simulink model "glucagon_model_ins"  (R2023b)
settings: Solver=VariableStepAuto  StartTime=0.0  StopTime=300  RelTol=1e-3
values from neighbouring files (symbols this model uses):
  GLUCAb = glucagon(1)    [glucamathins_main.m]
  KD = parameters(2)    [costfcnglumath.m]    (also in glucamathins_main.m = bestpar(2))
  kGLUCA = parameters(1)    [costfcnglumath.m]    (also in glucamathins_main.m = bestpar(1))
settings Model: Creator=Micaela  LastModifiedBy=Micaela
settings SolverCC: AlgebraicLoopSolver=TrustRegion
settings DataIOCC: ReturnWorkspaceOutputs=off
settings DebuggingCC: UnconnectedInputMsg=warning  UnconnectedOutputMsg=warning  UnconnectedLineMsg=warning  ArithmeticOperatorsInVariantConditions=warning
settings ModelReferenceCC: EnableRefExpFcnMdlSchedulingChecks=on
settings SFSimCC: SimUseLocalCustomCode=off  CustomCodeUndefinedFunction=UseInterfaceOnly
settings RTWCC: RTWUseLocalCustomCode=off

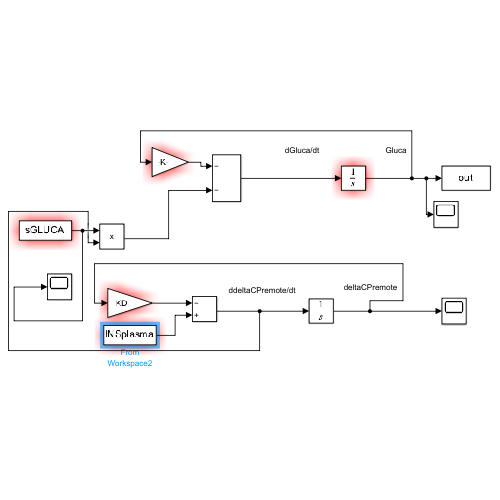
[thumbnail: Simulink's stored preview of the top-level diagram]
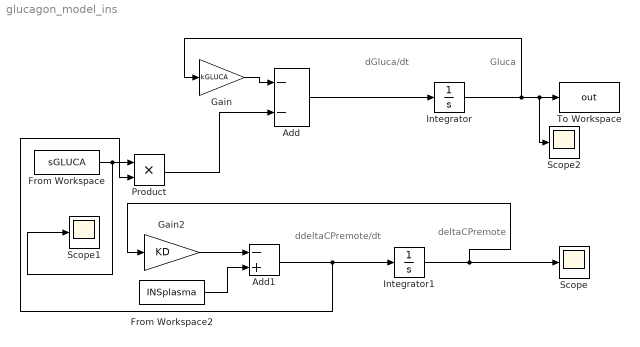
== system glucagon_model_ins ==
  note: deltaCPremote
  note: ddeltaCPremote/dt
  note: Gluca
  note: dGluca/dt
  Add : Sum  Inputs=--
  Add1 : Sum  Inputs=-+
  From Workspace : FromWorkspace  VariableName=sGLUCA
  From Workspace2 : FromWorkspace  VariableName=INSplasma
  Gain : Gain  Gain=kGLUCA
  Gain2 : Gain  Gain=KD
  Integrator : Integrator  InitialCondition=GLUCAb
  Integrator1 : Integrator
  Product : Product
  Scope : Scope
  Scope1 : Scope
  Scope2 : Scope
  To Workspace : ToWorkspace  VariableName=out  SaveFormat=Structure With Time  SampleTime=-1
  wires:
  Add/1 -> Integrator/1
  Integrator1/1 -> Scope/1, Gain2/1
  Gain/1 -> Add/1
  Integrator/1 -> Gain/1, Scope2/1, To Workspace/1
  From Workspace/1 -> Scope1/1, Product/1
  Add1/1 -> Product/2, Integrator1/1
  Gain2/1 -> Add1/1
  From Workspace2/1 -> Add1/2
  Product/1 -> Add/2
